simulink model "IEEE33BusTestSystem_DG_Control_IMC_nq3"  (R2019a)
settings: Solver=ode23t  StartTime=0.0  StopTime=20  FixedStep=5e-5  RelTol=1e-3
values from neighbouring files (symbols this model uses):
  du_n = 500    [IEEE33BusSystem_Control_Sim.m]    (also in IEEE33BusSystem_Control_Sim_nq3.m; IEEE33BusSystem_Control_Sim_nq5.m; IEEE33BusSystem_Ident.m; IEEE33BusSystem_Sim_compare.m)
  dy_n = 0.03    [IEEE33BusSystem_Control_Sim.m]    (also in IEEE33BusSystem_Control_Sim_nq3.m; IEEE33BusSystem_Control_Sim_nq5.m; IEEE33BusSystem_Ident.m; IEEE33BusSystem_Sim_compare.m)
  P_dg0 = 300*ones(1,6)    [IEEE33BusSystem_Control_Sim.m]    (also in IEEE33BusSystem_Control_Sim_nq3.m; IEEE33BusSystem_Control_Sim_nq5.m; IEEE33BusSystem_Ident.m; IEEE33BusSystem_op.m)
  P_dgf = 100*ones(1,6)    [IEEE33BusSystem_Control_Sim.m]    (also in IEEE33BusSystem_Control_Sim_nq3.m; IEEE33BusSystem_Control_Sim_nq5.m; IEEE33BusSystem_op.m = 300*ones(1,6); Kimc_d1_sce1-0.mat = [100 100 100 100 100 100])
  Q_dg0 = zeros(1,6)    [IEEE33BusSystem_Control_Sim.m]    (also in IEEE33BusSystem_Control_Sim_nq3.m; IEEE33BusSystem_Control_Sim_nq5.m; IEEE33BusSystem_Ident.m; IEEE33BusSystem_op.m)
  Tp = 500e-3    (= 0.5)    [IEEE33BusSystem.m]    (also in Kimc_d1_sce1-0.mat = 0.05; Kimc_d1_sce1-1.mat = 0.05; Kimc_d1_sce1-2.mat = 0.05; Kimc_d1_sce1-3.mat = 0.05)
  tPdg = 10*ones(1,6)    [IEEE33BusSystem_Control_Sim.m]    (also in IEEE33BusSystem_Control_Sim_nq3.m; IEEE33BusSystem_Control_Sim_nq5.m; IEEE33BusSystem_op.m = 0.5*ones(1,6); Kimc_d1_sce1-0.mat = [10 10 10 10 10 10])
  Tq = 50e-3    (= 0.05)    [IEEE33BusSystem.m]    (also in Kimc_d1_sce1-0.mat; Kimc_d1_sce1-1.mat; Kimc_d1_sce1-2.mat; Kimc_d1_sce1-3.mat)
  Ts = 0.005    [IEEE33BusSystem_Control_Sim.m]    (also in IEEE33BusSystem_Control_Sim_nq3.m; IEEE33BusSystem_Control_Sim_nq5.m; IEEE33BusSystem_Sim_compare.m = tout_d(2)-tout_d(1); IEEE33BusSystem_op.m)
  tsp = 3*ones(1,6)    [IEEE33BusSystem_Control_Sim.m]    (also in IEEE33BusSystem_Control_Sim_nq3.m; IEEE33BusSystem_Control_Sim_nq5.m; Kimc_d1_sce1-0.mat = [3 3 3 3 3 3]; Kimc_d1_sce1-1.mat = [3 3 3 3 3 3])
  v0 = ones(1,33)    [IEEE33BusSystem_Control_Sim.m]    (also in IEEE33BusSystem_Control_Sim_nq3.m; IEEE33BusSystem_Control_Sim_nq5.m; IEEE33BusSystem_Ident.m; IEEE33BusSystem_op.m)
  V_0 = v0_sim(CVs_sel)    [IEEE33BusSystem_Control_Sim.m]    (also in IEEE33BusSystem_Control_Sim_nq3.m = [v0_sim(14), v0_sim(18), v0_sim(21), v0_sim(25), v0_sim(30),; IEEE33BusSystem_Control_Sim_nq5.m = [v0_sim(14), v0_sim(18), v0_sim(21), v0_sim(25), v0_sim(30),; IEEE33BusSystem_Ident.m; IEEE33BusSystem_op.m = [v0(14), v0(18), v0(21), v0(25), v0(30), v0(33)])
  V_0_sp = [v0_sim(14), v0_sim(18), v0_sim(33)]    [IEEE33BusSystem_Control_Sim_nq3.m]    (also in IEEE33BusSystem_Control_Sim_nq5.m = [v0_sim(14), v0_sim(18), v0_sim(21), v0_sim(25), v0_sim(33)])
  Vsp = V_0    [IEEE33BusSystem_Control_Sim.m]    (also in IEEE33BusSystem_Control_Sim_nq3.m; IEEE33BusSystem_Control_Sim_nq5.m; Kimc_d1_sce1-0.mat = [0.9549 0.956 0.9966 0.9787 0.9486 0.9462]; Kimc_d1_sce1-1.mat = [0.9549 0.956 0.9966 0.9787 0.9486 0.9462])
libraries: powerlib x160, powerlib_meascontrol x33, cstblocks x2
(part 4 of 4)

== system IEEE33BusTestSystem_DG_Control_IMC_nq3/ADN/Measurements/Phasor RMS6 ==
  Vabc : Inport
  Sequence Analyzer (Phasor) : powerlib_meascontrol/Measurements/Sequence Analyzer (Phasor)  seq=Positive
      settings: SourceProductName=Simscape Power Systems  SourceProductBaseCode=PS
  Terminator : Terminator
  Vrms : Outport
  wires:
  Sequence Analyzer (Phasor)/1 -> Vrms/1
  Vabc/1 -> Sequence Analyzer (Phasor)/1
  Sequence Analyzer (Phasor)/2 -> Terminator/1

== system IEEE33BusTestSystem_DG_Control_IMC_nq3/ADN/Measurements/Phasor RMS7 ==
  Vabc : Inport
  Sequence Analyzer (Phasor) : powerlib_meascontrol/Measurements/Sequence Analyzer (Phasor)  seq=Positive
      settings: SourceProductName=Simscape Power Systems  SourceProductBaseCode=PS
  Terminator : Terminator
  Vrms : Outport
  wires:
  Sequence Analyzer (Phasor)/1 -> Vrms/1
  Vabc/1 -> Sequence Analyzer (Phasor)/1
  Sequence Analyzer (Phasor)/2 -> Terminator/1

== system IEEE33BusTestSystem_DG_Control_IMC_nq3/ADN/Measurements/Phasor RMS8 ==
  Vabc : Inport
  Sequence Analyzer (Phasor) : powerlib_meascontrol/Measurements/Sequence Analyzer (Phasor)  seq=Positive
      settings: SourceProductName=Simscape Power Systems  SourceProductBaseCode=PS
  Terminator : Terminator
  Vrms : Outport
  wires:
  Sequence Analyzer (Phasor)/1 -> Vrms/1
  Vabc/1 -> Sequence Analyzer (Phasor)/1
  Sequence Analyzer (Phasor)/2 -> Terminator/1

== system IEEE33BusTestSystem_DG_Control_IMC_nq3/ADN/Measurements/Phasor RMS9 ==
  Vabc : Inport
  Sequence Analyzer (Phasor) : powerlib_meascontrol/Measurements/Sequence Analyzer (Phasor)  seq=Positive
      settings: SourceProductName=Simscape Power Systems  SourceProductBaseCode=PS
  Terminator : Terminator
  Vrms : Outport
  wires:
  Sequence Analyzer (Phasor)/1 -> Vrms/1
  Vabc/1 -> Sequence Analyzer (Phasor)/1
  Sequence Analyzer (Phasor)/2 -> Terminator/1
